simulink model "doc_nonlinear_digital_demod"  (R2014a)
settings: Solver=VariableStepDiscrete  StartTime=0.0  StopTime=600  RelTol=1e-3
undefined symbols (not defined in the file or in its folder): gcbh, get, rcfiltgaincompat
libraries: commdigbbndcpm2 x2, commsink2 x2, commfilt2 x2, commchan3 x1, commrandsrc2 x1, dspsigops x1, commutil2 x1, simulink x1, dspstat3 x1
settings Model: Creator=The MathWorks Inc.
settings DataIOCC: SignalLoggingSaveFormat=ModelDataLogs
settings OptimizationCC: ExpressionDepthLimit=2147483647
settings DebuggingCC: UnderspecifiedInitializationDetection=Classic  FcnCallInpInsideContextMsg=UseLocalSettings  StateNameClashWarn=warning  StrictBusMsg=Warning
settings GRTTargetCC: CombineOutputUpdateFcns=off  GRTInterface=on

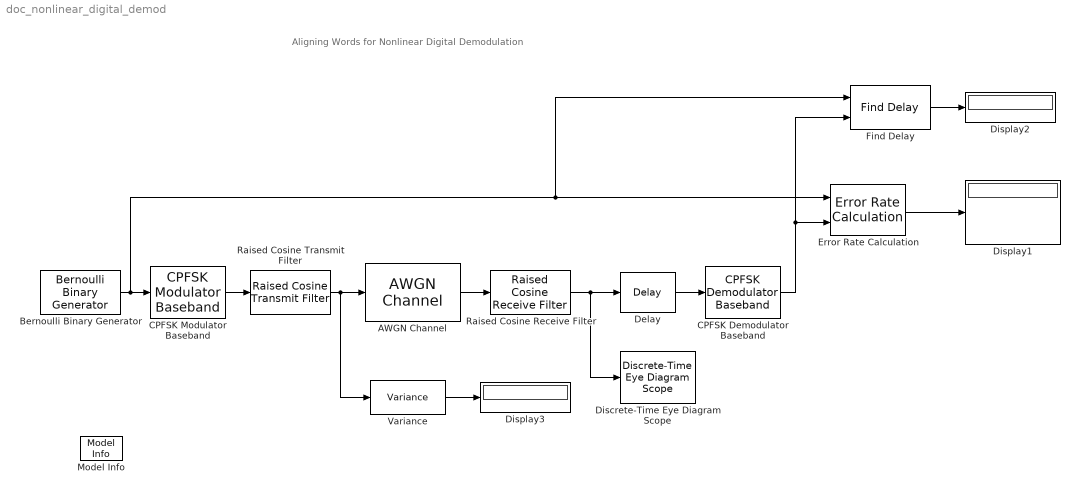
== system doc_nonlinear_digital_demod ==
  note: Aligning Words for Nonlinear Digital Demodulation
  AWGN Channel : commchan3/AWGN Channel  InputProcessing=Columns as channels (frame based)  seed=67  noiseMode="Signal to noise ratio  (Eb/No)"  EbNodB=5  EsNodB=10  SNRdB=10  bitsPerSym=1  Ps=0.1226  Tsym=1  variance=1
  Bernoulli Binary Generator : commrandsrc2/Bernoulli Binary Generator  P=0.5  seed=61  Ts=1  frameBased=off  sampPerFrame=1  orient=off  outDataType=double
  CPFSK Demodulator Baseband : commdigbbndcpm2/CPFSK Demodulator Baseband  Mnum=2  outputType=Bit  mappingType=Binary  modIdx=.5  phaseOffset=0  samplesPerSymbol=8  RateOptions=Allow multirate processing  traceBack=16  outDtype=double
  CPFSK Modulator Baseband : commdigbbndcpm2/CPFSK Modulator Baseband  Mnum=2  inputType=Bit  mappingType=Binary  modIdx=.5  phaseOffset=0  samplesPerSymbol=8  RateOptions=Allow multirate processing  outDataType=double
  Delay : dspsigops/Delay  dly_unit=Samples  delay=8  ic_detail=off  dif_ic_for_ch=off  dif_ic_for_dly=off  ic=0  reset_popup=None
  Discrete-Time Eye Diagram Scope : commsink2/Discrete-Time Eye Diagram Scope  Tag=EyeDiagram  sampPerSymb=8  offsetEye=0  symbPerTrace=1  numTraces=40  numNewFrames=10  LineStyles=-  LineColors=b  dupPoints=on  fading=on  render=on  AxisGrid=on  yMin=-4.38100164960216  yMax=4.11454633354114  inphaseLabel=In-phase Amplitude  quadratureLabel=Quadrature Amplitude  openScopeAtSimStart=off  dispDiagram=In-phase and Quadrature  FrameNumber=off  FigPos=get(0,'defaultfigureposition');  figTitle=Eye Diagram  block_type_=eye  numLinesMax=8
  Display1 : Display
  Display2 : Display
  Display3 : Display
  Error Rate Calculation : commsink2/Error Rate Calculation  N=17+2  st_delay=0  cp_mode=Entire frame  subframe=[]  PMode=Port  WsName=ErrorVec  RsMode2=off  stop=off  numErr=100  maxBits=1e6
  Find Delay : commutil2/Find Delay  corrLength=200  chgSigOP=off  stopUpdate=off  numConstDelay=3
  Model Info : simulink/Model-Wide Utilities/Model Info  InitialBlockCM=None  BlockCM=None  Frame=on  DisplayStringWithTags=Info  HorizontalTextAlignment=Center  LeftAlignmentValue=0.5  SourceBlockDiagram=doc_nonlinear_digital_demod  TagMaxNumber=20
  Raised Cosine Receive Filter : commfilt2/Raised Cosine Receive Filter  filtType=Square root  N=8  filtSpan=2*(4)  currentFiltSpan=2*(4)  D=4  R=0.2  sampMode=Mute  saveAsFlag=0  rateMode=Downsampling  downFactor=8  downOffset=0  framing=Maintain input frame size  checkGain=Normalized  filterGain=rcfiltgaincompat(gcbh)  checkCoeff=on  variableName=rcRxFilt1  launchFVT=off  roundingMode=Floor  overflowMode=off
  Raised Cosine Transmit Filter : commfilt2/Raised Cosine Transmit Filter  filtType=Square root  filtSpan=2*(4)  currentFiltSpan=2*(4)  D=4  R=0.2  sampMode=Mute  saveAsFlag=0  N=8  framing=Maintain input frame size  checkGain=Normalized  filterGain=rcfiltgaincompat(gcbh)  checkCoeff=off  variableName=rcTxFilt  launchFVT=off  roundingMode=Floor  overflowMode=off
  Variance : dspstat3/Variance  run=on  reset_popup=None  directionMode=Each column  dimension=1  treatSBRowAsCol=on  roiEnable=off  roiType=Rectangles  roiPortion=Entire ROI  roiOutput=Individual statistics for each ROI  roiFlag=off  roundingMode=Floor  overflowMode=off
  wires:
  Bernoulli Binary Generator/1 -> CPFSK Modulator Baseband/1, Error Rate Calculation/1, Find Delay/1
  CPFSK Modulator Baseband/1 -> Raised Cosine Transmit Filter/1
  Raised Cosine Transmit Filter/1 -> AWGN Channel/1, Variance/1
  AWGN Channel/1 -> Raised Cosine Receive Filter/1
  Raised Cosine Receive Filter/1 -> Delay/1, Discrete-Time Eye Diagram Scope/1
  Delay/1 -> CPFSK Demodulator Baseband/1
  Find Delay/1 -> Display2/1
  Error Rate Calculation/1 -> Display1/1
  Variance/1 -> Display3/1
  CPFSK Demodulator Baseband/1 -> Find Delay/2, Error Rate Calculation/2
